simulink model "sim_ex_4link_rel_basic"  (R2016a)
settings: Solver=FixedStepAuto  StartTime=0.0  StopTime=0.4  FixedStep=0.002  RelTol=1e-3
model workspace: external: MAT-File (data not in the file)
values from neighbouring files (symbols this model uses):
  desire = [6*pi/12+pi/9;-10/6*pi;pi/3;-2*pi/18]    [algorithm2.m]    (also in algorithm3.m = [6*pi/12+pi/18;-10/6*pi;pi/3;-2*pi/18]; algorithm4.m; cyclic.m; desire_test.m = [6*pi/12+pi/18;-3/2*pi;pi/3;-2*pi/18])
  dgain = [24;24;24;24]    [algorithm2.m]    (also in algorithm3.m; algorithm4.m = 3*[24;24;24;24]; cyclic.m = 4*[24;24;24;24]; desire_test.m)
  ini = [3/4*pi; -1/4*pi; 1/12*pi; -1/3*pi; 0;0;0;0]    [algorithm2.m]    (also in algorithm3.m; algorithm4.m; cyclic.m; desire_test.m)
  pgain = 1/4*[dgain(1)^2;dgain(2)^2;dgain(3)^2;dgain(4)^2]    [algorithm2.m]    (also in algorithm3.m; algorithm4.m; cyclic.m; desire_test.m)
settings Model: Creator=HYUNSOO  LastModifiedBy=Home
settings DataIOCC: LimitDataPoints=on  SaveFormat=Array
settings DebuggingCC: UnderspecifiedInitializationDetection=Classic  MergeDetectMultiDrivingBlocksExec=none  SolverPrmCheckMsg=warning  AllowSymbolicDim=off  StateNameClashWarn=warning
settings HardwareCC: ProdBitPerPointer=32  ProdLargestAtomicFloat=None  ProdIntDivRoundTo=Undefined  ProdEndianess=Unspecified  ProdWordSize=32  ProdHWDeviceType=32-bit Generic
settings ModelReferenceCC: PropagateSignalLabelsOutOfModel=off
settings ConfigComp: CovModelRefEnable=Off

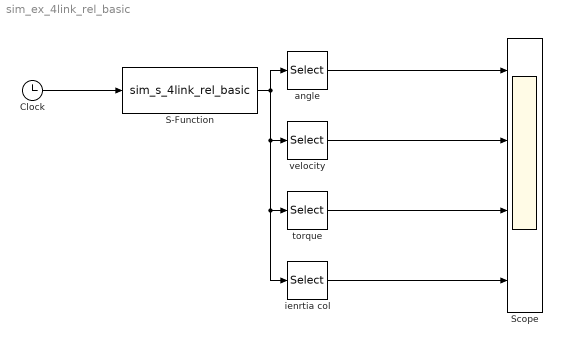
== system sim_ex_4link_rel_basic ==
  Clock : Clock
  S-Function : S-Function  FunctionName=sim_s_4link_rel_basic  Parameters=dgain,pgain,desire,ini  SFunctionDeploymentMode=off  EnableBusSupport=off
  Scope : Scope  NumInputPorts=4
  angle : Selector  InputPortWidth=15  IndexOptions=Index vector (dialog)  Indices=[1 2 3 4]  OutputSizes=1
  ienrtia col : Selector  InputPortWidth=15  IndexOptions=Index vector (dialog)  Indices=[12 13 14 15]  OutputSizes=1
  torque : Selector  InputPortWidth=15  IndexOptions=Index vector (dialog)  Indices=[9 10 11]  OutputSizes=1
  velocity : Selector  InputPortWidth=15  IndexOptions=Index vector (dialog)  Indices=[5 6 7 8]  OutputSizes=1
  wires:
  Clock/1 -> S-Function/1
  S-Function/1 -> ienrtia col/1, torque/1, velocity/1, angle/1
  angle/1 -> Scope/1
  velocity/1 -> Scope/2
  torque/1 -> Scope/3
  ienrtia col/1 -> Scope/4
